simulink model "ADCTestSim1"  (R2020b)
settings: Solver=VariableStepAuto  StartTime=0.0  StopTime=4  RelTol=1e-3
libraries: fl_lib x8, nesl_utility x3
settings Model: Creator=Miodrag Bolic  LastModifiedBy=dhrumilnaik
settings DataIOCC: ReturnWorkspaceOutputs=off
settings DebuggingCC: ArithmeticOperatorsInVariantConditions=warning
settings SFSimCC: CustomCodeUndefinedFunction=UseInterfaceOnly

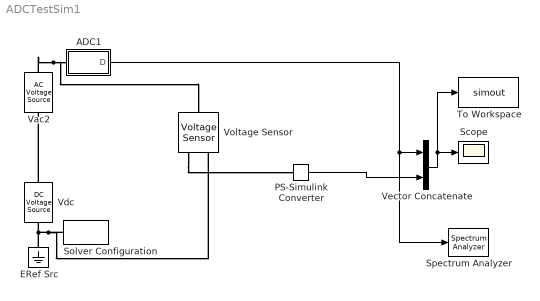
== system ADCTestSim1 ==
  " Scope" : Scope
  ADC1 : Subsystem  mask(ADC){fs=12, N=4, vmax=5, ileak=1e-9, C=10e-12}
      mask prompts: fs "Sampling rate (Hz)"; N "Number of bits"; vmax "Input voltage for max output (V)"; ileak "Leakage current (A)"; C "Pin capacitance (F)"
      mask help: Simplified analog-to-digital converter
  ERef Src : fl_lib/Electrical/Electrical Elements/Electrical Reference
      settings: SourceProductName=Foundation Library
  PS-Simulink Converter : nesl_utility/PS-Simulink Converter  PhysicalDomain=network_engine_domain  SubClassName=ps_output  LeftPortType=input  RightPortType=output  PseudoPeriodic=off  Frequencies=[]  Unit=1  AffineConversion=off
  Solver Configuration : nesl_utility/Solver Configuration  PhysicalDomain=network_engine_domain  SubClassName=solver  LeftPortType=input  RightPortType=generic  Tones=[]  Harmonics=[]  SimulateNoise=off  Profile=off  UseLocalSampling=off  EnableSwitchedLinearOptims=on  FrequencyDomain=off  UseCCode=off  RelTol=0.001  AbsTol=1e-06  MinStep=1e-09  ToWorkspace=off  RevertToSquareIcSolve=off  NumHomotopyIterations=100  PhasorMode=off  PhasorModeNumHarmonics=1  DoDC=off  ResidualTolerance=1e-9  UseLocalSolver=off  LocalSolverChoice=NE_BACKWARD_EULER_ADVANCER  LocalSolverSampleTime=1e-6  DoFixedCost=off  MaxNonlinIter=3  MaxModeIter=2  ComputeImpulses=off  ImpulseIterations=2  LinearAlgebra=auto  EquationFormulation=NE_TIME_EF  DelaysMemoryBudget=1024  AutomaticFiltering=on  FilteringTimeConstant=0.001  PartitionStorageMethod=AS_NEEDED  PartitionMemoryBudget=1024  PartitionMethod=FAST
  Spectrum Analyzer : SpectrumAnalyzer  Tag=Scope
  To Workspace : ToWorkspace  VariableName=simout  SaveFormat=Timeseries  SampleTime=0.001
  Vac2 : fl_lib/Electrical/Electrical Sources/AC Voltage Source  amp=1 V  shift=0 deg  frequency=0.25 Hz  omega=0 rad/s
      settings: SourceProductName=Foundation Library
      settings: AttributesFormatString=|
      | %<amp> %<amp_unit>
      | %<frequency> %<frequency_unit>
  Vdc : fl_lib/Electrical/Electrical Sources/DC Voltage Source  v0=1.5 V
      settings: AttributesFormatString=%<v0> %<v0_unit>  SourceProductName=Foundation Library
  Vector Concatenate : Concatenate  Mode=Multidimensional array  ConcatenateDimension=2
  Voltage Sensor : fl_lib/Electrical/Electrical Sensors/Voltage Sensor
  wires:
  ADC1/1(D) -> Vector Concatenate/1, Spectrum Analyzer/1
  Vector Concatenate/1 -> To Workspace/1, " Scope"/1
  PS-Simulink Converter/1 -> Vector Concatenate/2
  connections:
  Solver Configuration/RConn1 -- Vdc/RConn1 -- ERef Src/LConn1 -- Voltage Sensor/RConn2
  Vac2/LConn1 -- Voltage Sensor/LConn1 -- ADC1/LConn1
  Vdc/LConn1 -- Vac2/RConn1
  Voltage Sensor/RConn1 -- PS-Simulink Converter/LConn1

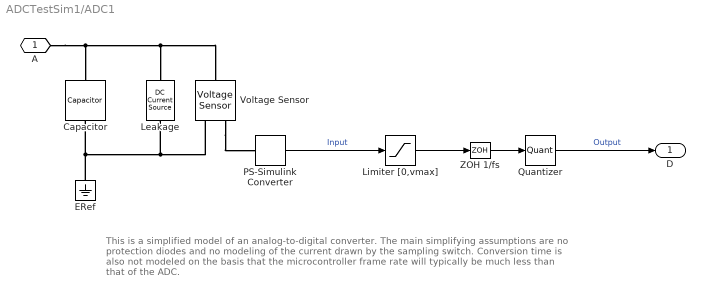
== system ADCTestSim1/ADC1 ==
  note: This is a simplified model of an analog-to-digital converter. The main simplifying assumptions
      | are no protection diodes and no modeling of the current drawn by the sampling switch.
      | Conversion time is also not modeled on the basis that the microcontroller frame rate will
      | typically be much less than that of the ADC.
  Capacitor : fl_lib/Electrical/Electrical Elements/Capacitor  c=1e-6 F  r=1e-6 Ohm  g=0 1/Ohm  i_specify=off  i_priority=High  i=0 A  i_nominal_specify=off  i_nominal_unit=A  i_nominal_value=1  v_specify=off  v_priority=High  v=0 V  v_nominal_specify=off  v_nominal_unit=V  v_nominal_value=1  vc_specify=on  vc_priority=High  vc=0 V  vc_nominal_specify=off  vc_nominal_unit=V  vc_nominal_value=1
      settings: SourceProductName=Foundation Library
  ERef : fl_lib/Electrical/Electrical Elements/Electrical Reference
      settings: SourceProductName=Foundation Library
  Leakage : fl_lib/Electrical/Electrical Sources/DC Current Source  i0=ileak A
      settings: SourceProductName=Foundation Library  InternalSimscapePortConfiguration="{\"Bottom\":[],\"Left\":[{\"id\":\"p\",\"label\":\"\",\"type\":\"foundation.electrical.electrical\"}],\"Right\":[{\"id\":\"n\",\"label\":\"\",\"type\":\"foundation.electrical.electrical\"}],\"Top\":[]}"
  Limiter [0,vmax] : Saturate  UpperLimit=vmax  LowerLimit=0
  PS-Simulink Converter : nesl_utility/PS-Simulink Converter  PhysicalDomain=network_engine_domain  SubClassName=ps_output  LeftPortType=input  RightPortType=output  PseudoPeriodic=off  Frequencies=[]  Unit=V  AffineConversion=off
  Quantizer : Quantizer  QuantizationInterval=vmax/2^N
  Voltage Sensor : fl_lib/Electrical/Electrical Sensors/Voltage Sensor
      settings: SourceProductName=Foundation Library
  ZOH 1/fs : ZeroOrderHold  SampleTime=1/fs
  A : PMIOPort  Side=Left
  D : Outport  VectorParamsAs1DForOutWhenUnconnected=off
  wires:
  PS-Simulink Converter/1 -> Limiter [0,vmax]/1  "Input"
  Limiter [0,vmax]/1 -> ZOH 1/fs/1
  Quantizer/1 -> D/1  "Output"
  ZOH 1/fs/1 -> Quantizer/1
  connections:
  A/RConn1 -- Voltage Sensor/LConn1 -- Leakage/RConn1 -- Capacitor/LConn1
  ERef/LConn1 -- Voltage Sensor/RConn2 -- Leakage/LConn1 -- Capacitor/RConn1
  Voltage Sensor/RConn1 -- PS-Simulink Converter/LConn1
